simulink model "atrias_HW_boom_nmSt_kinSw_v4"  (R2015a)
settings: Solver=ode4  StartTime=0.0  StopTime=inf  FixedStep=sample_time  RelTol=1e-3
values from neighbouring files (symbols this model uses):
  control_start_time = 15    [setParams.m]
  flag_CtrlMode = 0    [setParams.m]
  kinSw_alpha_start = 130*pi/180    (= 2.26892802759)    [setParams.m]
  kinSw_alpha_tgt = 70*pi/180    (= 1.2217304764)    [setParams.m]
  kinSw_t_start = 0.5    [setParams.m]
  poser_LLegAlp = (initial_l_leg_angle -pi/2)*180/pi    (= 105)    [setParams.m]
  poser_LLegLen = initial_l_leg_length    (= 0.8)    [setParams.m]
  poser_RLegAlp = (initial_r_leg_angle -pi/2)*180/pi    (= 75)    [setParams.m]
  poser_RLegLen = initial_r_leg_length    (= 0.8)    [setParams.m]
  tune_kinSw_alpha_start = kinSw_alpha_start*180/pi    (= 130)    [setParams.m]
  tune_kinSw_alpha_tgt = kinSw_alpha_tgt*180/pi    (= 70)    [setParams.m]
  tune_kinSw_gClr_tgt = kinSw_gClr    (= 0.15)    [setParams.m]
  tune_kinSw_gH_tgt = kinSw_gH_tgt    (= -0.01)    [setParams.m]
  tune_M1_G = 9.5    [setParams.m]
  tune_M3_0 = CtrlPar_theta0*180/pi    [setParams.m]
  tune_M3_D = St_GainDTh_HFL*5    [setParams.m]
  tune_M3_P = St_GainTh_HFL*5    [setParams.m]
  tune_M4_G = 1    [setParams.m]
undefined symbols (not defined in the file or in its folder): A1_notch_f1, A2_notch_f1, A_kalman_fourbar_gear, A_lpf_dtau, B1_lpf_dtau, B1_notch_f1, B2_lpf_dtau, B2_notch_f1, B_kalman_fourbar_gear, boom_mount_angle, boom_mount_to_center_diagonal, c_jointstop, C_kalman_fourbar_gear, contactThr, d_vertical_com, delta_phi_max, delta_phi_max_buffer, delta_phi_max_dropoff, delta_phi_min, Discrete, FmaxBFSH, FmaxGLU, FmaxHAM, FmaxHFL, FmaxRF, FmaxVAS, FPCtrlPar, g, gain_nodes_sea_torque, HIP_MTR_MAX_CONT_TORQUE, initial_dx_estimate, j_motor, k_leg_spring, K_notch_f1, k_sea, kalman_load_to_deflect_transmission, kd_lateral, kd_motor, kd_shin_max, kd_shin_min, kd_splay_max, kd_splay_min, kd_thigh_max, kd_thigh_min, kp_lateral, kp_motor, kp_sea_torque, kp_shin_max, kp_shin_min, kp_splay_max, kp_splay_min, kp_thigh_max, kp_thigh_min, l_boom, l_seg, l_v, lateral_motor_efficiency, lateral_offset, lateral_target_angle_right, lateral_transition_force ... (+123)
libraries: simulink_extras x28, simulink x11, ctrlSharedLib x4
(part 1 of 8)
settings Model: CovSFcnEnable=off  Creator=wmartin  LastModifiedBy=smsong
settings SolverCC: EnableConcurrentExecution=on
settings DataIOCC: LimitDataPoints=off  MaxDataPoints=1000000000  SaveFormat=StructureWithTime  SignalLogging=off  DSMLogging=off  VisualizeSimOutput=off
settings OptimizationCC: BlockReduction=off  OptimizeBlockIOStorage=off  BufferReuse=off  GlobalBufferReuse=off  ExpressionFolding=off  ExpressionDepthLimit=2147483647  LocalBlockOutputs=off  SimCompilerOptimization=on
settings DebuggingCC: UnderspecifiedInitializationDetection=Classic  MergeDetectMultiDrivingBlocksExec=none  SolverPrmCheckMsg=warning  StateNameClashWarn=warning
settings HardwareCC: ProdIntDivRoundTo=Zero  ProdEndianess=LittleEndian  ProdLongLongMode=on  ProdHWDeviceType=Generic->32-bit x86 compatible
settings ModelReferenceCC: UpdateModelReferenceTargets=IfOutOfDate  ModelReferenceNumInstancesAllowed=Single  ModelReferenceMinAlgLoopOccurrences=on
settings RTWCC: SystemTargetFile=slrt.tlc  TemplateMakefile=slrt_default_tmf  Description=Simulink Real-Time  RTWVerbose=off  RTWCompilerOptimization=on
settings CodeAppCC: MaxIdLength=256
settings SimulinkRealTimeCC: GeneratePreprocessorConditionals=Disable all  RL32LogBufSizeModifier=1e8

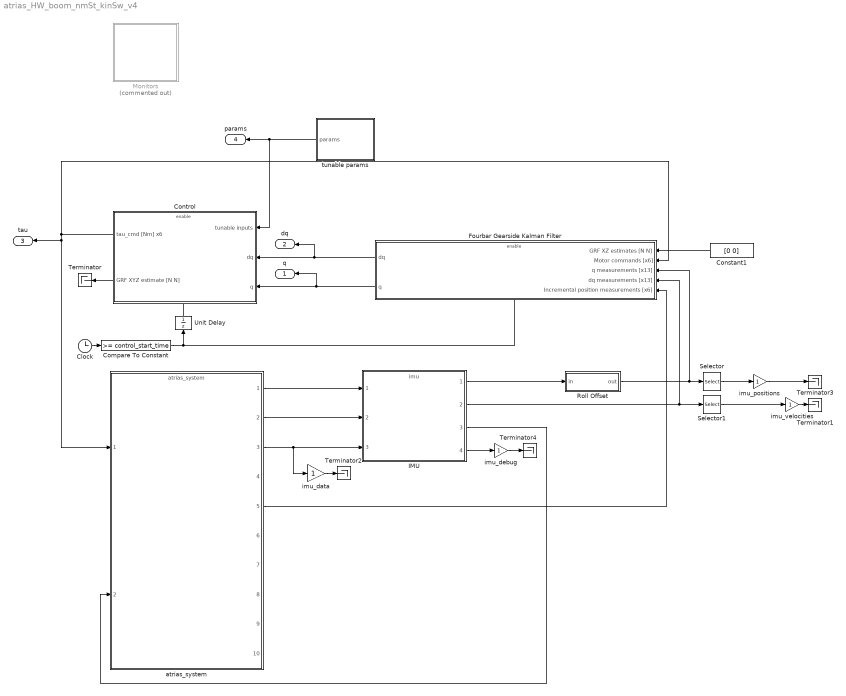
== system atrias_HW_boom_nmSt_kinSw_v4 ==
  Clock : Clock
  Compare To Constant : simulink/Logic and Bit Operations/Compare To Constant  relop=>=  const=control_start_time  OutDataTypeStr=boolean
  Constant1 : Constant  Value=[0 0]
  Control : Subsystem
  Fourbar Gearside Kalman Filter : Subsystem
  IMU : ModelReference  ModelNameDialog=imu  SimulationMode=Normal  ModelReferenceVersion=1.2453  CopyOfModelName=imu  DefaultDataLogging=on
  Monitors : Subsystem  Commented=on
  Roll Offset : Subsystem
  Selector : Selector  InputPortWidth=13  Indices=[11 12 13]
  Selector1 : Selector  InputPortWidth=13  Indices=[11 12 13]
  Terminator{,1..4} (5 alike) : Terminator
  Unit Delay : UnitDelay  SampleTime=-1
  atrias_system : ModelReference  ModelNameDialog=atrias_system  SimulationMode=Normal  ModelReferenceVersion=1.2798  CopyOfModelName=atrias_system  DefaultDataLogging=on
  imu_data : Gain
  imu_debug : Gain
  imu_positions : Gain
  imu_velocities : Gain
  tunable params : Subsystem
  q : Outport
  dq : Outport  Port=2
  tau : Outport  Port=3
  params : Outport  Port=4
  wires:
  Clock/1 -> Compare To Constant/1
  Compare To Constant/1 -> Fourbar Gearside Kalman Filter/Enable, Unit Delay/1
  imu_data/1 -> Terminator2/1
  imu_velocities/1 -> Terminator1/1
  imu_positions/1 -> Terminator3/1
  imu_debug/1 -> Terminator4/1
  IMU/4 -> imu_debug/1
  Selector/1 -> imu_positions/1
  Selector1/1 -> imu_velocities/1
  atrias_system/1 -> IMU/1
  IMU/2 -> Fourbar Gearside Kalman Filter/4(dq measurements [x13]), Selector1/1
  IMU/1 -> Roll Offset/1(in)
  Control/1(tau_cmd [Nm] x6) -> atrias_system/1, tau/1, Fourbar Gearside Kalman Filter/2(Motor commands [x6])
  atrias_system/2 -> IMU/2
  atrias_system/3 -> imu_data/1, IMU/3
  IMU/3 -> atrias_system/2
  Unit Delay/1 -> Control/Enable
  Control/2(GRF XYZ estimate [N N]) -> Terminator/1
  Fourbar Gearside Kalman Filter/1(dq) -> dq/1, Control/2(dq)
  Fourbar Gearside Kalman Filter/2(q) -> q/1, Control/3(q)
  atrias_system/5 -> Fourbar Gearside Kalman Filter/5(Incremental position measurements [x6])
  Constant1/1 -> Fourbar Gearside Kalman Filter/1(GRF XZ estimates [N N])
  Roll Offset/1(out) -> Fourbar Gearside Kalman Filter/3(q measurements [x13]), Selector/1
  tunable params/1(params) -> params/1, Control/1(tunable inputs)

== system atrias_HW_boom_nmSt_kinSw_v4/Control ==
  tunable inputs : Inport
  dq : Inport  Port=2
  q : Inport  Port=3
  Enable : EnablePort  StatesWhenEnabling=reset  PropagateVarSize=During execution
  Actuator Control : Subsystem
  Behavior Control : Subsystem
  Control Switch : Subsystem
  Poser : Subsystem
  Tunable Control Parameters : Subsystem
  tau_cmd [Nm] x6 : Outport  InitialOutput=[0 0 0 0 0 0]
  GRF XYZ estimate [N N] : Outport  Port=2  InitialOutput=[0 0 0]
  wires:
  q/1 -> Behavior Control/2(q [rad] x13), Actuator Control/4(q)
  dq/1 -> Behavior Control/1(dq [rad/s] x13), Actuator Control/5(dq)
  Actuator Control/1(tau_cmd [Nm] x6) -> tau_cmd [Nm] x6/1
  Behavior Control/4(GRF XYZ estimates [N N N]) -> GRF XYZ estimate [N N]/1
  tunable inputs/1 -> Tunable Control Parameters/1(tunable inputs)
  Control Switch/3(Force / Position Control [1/0] x4) -> Actuator Control/3(Enable SEA Control [1/0] x4)
  Control Switch/2(SEA Torque Velocity Command [Nm] x4) -> Actuator Control/2(Desired SEA Torque Velocity [Nm] x4)
  Control Switch/1(Motor Torque Command [Nm] x6) -> Actuator Control/1(Desired Torque [Nm] x6)
  Poser/1(Motor Torque Command [Nm] x6) -> Control Switch/1(Pose Comm [Nm] x6)
  Poser/2(SEA Torque Velocity Command [Nm] x4) -> Control Switch/2(Pose Comm [Nm] x4)
  Poser/3(Force / Position Control [1/0] x4) -> Control Switch/3(Pose Comm [1/0] x4)
  Behavior Control/1(Motor Torque Command [Nm] x6) -> Control Switch/4(NM Comm [Nm] x6)
  Behavior Control/2(SEA Torque Velocity Command [Nm] x4) -> Control Switch/5(NM Comm [Nm] x4)
  Behavior Control/3(Force / Position Control [1/0] x4) -> Control Switch/6(NM Comm [1/0] x4)

== system atrias_HW_boom_nmSt_kinSw_v4/Fourbar Gearside Kalman Filter ==
  note: Order:
      | rightBack
      | rightFront
      | leftBack
      | leftFront
  GRF XZ estimates [N N] : Inport  SampleTime=sample_time
  Motor commands [x6] : Inport  Port=2  SampleTime=sample_time
  q measurements [x13] : Inport  Port=3  SampleTime=sample_time
  dq measurements [x13] : Inport  Port=4  SampleTime=sample_time
  Incremental position measurements [x6] : Inport  Port=5  SampleTime=sample_time
  Enable : EnablePort  ShowOutputPort=on
  Covariance Estimates : MATLAB Function  TreatAsAtomicUnit=on
  Demux{,1..4} (5 alike) : Demux
  Demux{5..8} (4 alike) : Demux  Outputs=2
  External Trunk Torque Estimate : MATLAB Function  TreatAsAtomicUnit=on
  Fourbar Gear Kalman Filter {1..4} (4 alike) : ctrlSharedLib/Kalman Filter  TimeDomain=Discrete-Time  UseCurrentEstimator=on  ModelSource=Individual A, B, C, D matrices  ModelSourceVariable=A_kf  A=A_kalman_fourbar_gear  B=B_kalman_fourbar_gear  C=C_kalman_fourbar_gear  D=0  NumberOfStates=2  NumberOfInputs=1  NumberOfOutputs=2  InitialEstimateSource=Input port  X0=initial_dx_estimate  P0=P0_kalman_transverse  UseK=off  UseGH=on  NumberOfProcessNoiseInputs=1  G=G_kalman_fourbar_gear  TimeInvariantG=on  H=0  TimeInvariantH=on  Q=1  TimeInvariantQ=off  R=1  TimeInvariantR=off  N=0  TimeInvariantN=on  AddInputPort=on  AddEnablePort=off  ExternalReset=Either  OutputEstimatedY=off  OutputP=on  Ts=sample_time
  Mux{,3,7..9,11,13,15,17..18} (10 alike) : Mux  Inputs=2
  Mux{1,4..6,16} (5 alike) : Mux
  Mux{2,10,12,14} (4 alike) : Mux  Inputs=3
  P0_kalman_fourbar_gear{,1..3} (4 alike) : Constant  Value=P0_kalman_fourbar_gear
  Selector : Selector  InputPortWidth=17  Indices=[1 14 3 15 5 16 7 17 9 10 11 12 13]
  Selector1 : Selector  InputPortWidth=17  Indices=[1 14 3 15 5 16 7 17 9 10 11 12 13]
  Spring Stiffness 1 : Gain  Gain=k_sea
  Spring Stiffness 2 : Gain  Gain=1/LEG_MTR_GEAR_RATIO
  Sum : Sum  Inputs=-|+
  Terminator : Terminator
  Terminator1 : Terminator
  Terminator2 : Terminator
  Unit Delay{,1..9} (10 alike) : UnitDelay  SampleTime=-1
  Zero-Order Hold : ZeroOrderHold  SampleTime=sample_time
  eigen values 1 : MATLAB Function  TreatAsAtomicUnit=on
  eigen values 2 : MATLAB Function  TreatAsAtomicUnit=on
  eigen values 3 : MATLAB Function  TreatAsAtomicUnit=on
  "eigen values4 " : MATLAB Function  TreatAsAtomicUnit=on
  kalman_filtered_position : Gain
  kalman_filtered_velocity : Gain
  kalman_uncertainty : Gain
  select absolute relative gear position : Selector  InputPortWidth=13  Indices=[2 4 6 8]
  select absolute relative gear velocity : Selector  InputPortWidth=13  Indices=[2 4 6 8]
  select absolute relative load position : Selector  InputPortWidth=13  Indices=[2 4 6 8]
  select fourbar motors : Selector  InputPortWidth=6  Indices=[1 2 3 4]
  select incremental relative gear position : Selector  InputPortWidth=6  Indices=[1 2 3 4]
  select torso pitch : Selector  InputPortWidth=13  Indices=[13]
  select_position{1,3,5,7} (4 alike) : Selector  NumberOfDimensions=2  InputPortWidth=2  IndexOptions=Index vector (dialog),Index vector (dialog)  Indices=[1],[1]  OutputSizes=1,1
  dq : Outport
  q : Outport  Port=2
  wires:
  select incremental relative gear position/1 -> Demux/1
  q measurements [x13]/1 -> select absolute relative gear position/1, Mux17/1, select absolute relative load position/1, select torso pitch/1
  Incremental position measurements [x6]/1 -> select incremental relative gear position/1
  Motor commands [x6]/1 -> Unit Delay8/1
  select fourbar motors/1 -> Spring Stiffness 2/1
  P0_kalman_fourbar_gear/1 -> Fourbar Gear Kalman Filter 1/4
  Mux/1 -> Fourbar Gear Kalman Filter 1/3
  select absolute relative gear velocity/1 -> Demux3/1
  dq measurements [x13]/1 -> Mux18/1, select absolute relative gear velocity/1
  Demux3/1 -> Mux/2
  GRF XZ estimates [N N]/1 -> Unit Delay9/1
  Spring Stiffness 1/1 -> Demux4/1, External Trunk Torque Estimate/3(spring_torque), Covariance Estimates/1(spring_torque)
  Fourbar Gear Kalman Filter 1/1 -> Unit Delay/1
  Demux5/1 -> Mux1/1, Mux5/1
  Mux1/1 -> Sum/2, Mux17/2, kalman_filtered_position/1
  select absolute relative load position/1 -> Sum/1
  Sum/1 -> Spring Stiffness 1/1
  External Trunk Torque Estimate/1(tau_trunk) -> Mux2/3, Mux10/3, Mux12/3, Mux14/3
  Demux4/1 -> Mux2/1
  Demux2/1 -> Mux2/2
  Mux2/1 -> Fourbar Gear Kalman Filter 1/1
  Demux/1 -> Mux3/2
  Demux1/1 -> Mux3/1, Mux/1
  Mux3/1 -> Fourbar Gear Kalman Filter 1/2
  Fourbar Gear Kalman Filter 1/2 -> Unit Delay1/1
  Mux4/1 -> Covariance Estimates/4(state_uncertainty)
  select absolute relative gear position/1 -> Covariance Estimates/2(absolute_gear), Demux1/1
  Mux5/1 -> Covariance Estimates/3(current_position_estimate)
  Covariance Estimates/1(Q1) -> Fourbar Gear Kalman Filter 1/6
  Covariance Estimates/2(R1) -> Fourbar Gear Kalman Filter 1/7
  select torso pitch/1 -> External Trunk Torque Estimate/4(torso_pitch)
  select_position1/1 -> Mux4/1
  P0_kalman_fourbar_gear1/1 -> Fourbar Gear Kalman Filter 2/4
  Fourbar Gear Kalman Filter 2/1 -> Unit Delay2/1
  Fourbar Gear Kalman Filter 2/2 -> Unit Delay3/1
  P0_kalman_fourbar_gear2/1 -> Fourbar Gear Kalman Filter 3/4
  Fourbar Gear Kalman Filter 3/1 -> Unit Delay4/1
  Fourbar Gear Kalman Filter 3/2 -> Unit Delay5/1
  P0_kalman_fourbar_gear3/1 -> Fourbar Gear Kalman Filter 4/4
  Fourbar Gear Kalman Filter 4/1 -> Unit Delay6/1
  Fourbar Gear Kalman Filter 4/2 -> Unit Delay7/1
  Covariance Estimates/3(Q2) -> Fourbar Gear Kalman Filter 2/6
  Covariance Estimates/5(Q3) -> Fourbar Gear Kalman Filter 3/6
  Covariance Estimates/7(Q4) -> Fourbar Gear Kalman Filter 4/6
  Covariance Estimates/4(R2) -> Fourbar Gear Kalman Filter 2/7
  Covariance Estimates/6(R3) -> Fourbar Gear Kalman Filter 3/7
  Covariance Estimates/8(R4) -> Fourbar Gear Kalman Filter 4/7
  select_position3/1 -> Mux4/2
  select_position5/1 -> Mux4/3
  select_position7/1 -> Mux4/4
  Demux6/1 -> Mux5/2, Mux1/2
  Demux7/1 -> Mux1/3, Mux5/3
  Demux8/1 -> Mux1/4, Mux5/4
  kalman_filtered_position/1 -> Terminator/1
  Enable/1 -> Zero-Order Hold/1
  Mux7/1 -> Fourbar Gear Kalman Filter 2/3
  Mux8/1 -> Fourbar Gear Kalman Filter 3/3
  Mux9/1 -> Fourbar Gear Kalman Filter 4/3
  Mux10/1 -> Fourbar Gear Kalman Filter 2/1
  Mux11/1 -> Fourbar Gear Kalman Filter 2/2
  Mux13/1 -> Fourbar Gear Kalman Filter 3/2
  Mux12/1 -> Fourbar Gear Kalman Filter 3/1
  Mux15/1 -> Fourbar Gear Kalman Filter 4/2
  Mux14/1 -> Fourbar Gear Kalman Filter 4/1
  Demux3/2 -> Mux7/2
  Demux3/3 -> Mux8/2
  Demux3/4 -> Mux9/2
  Demux1/2 -> Mux7/1, Mux11/1
  Demux1/3 -> Mux13/1, Mux8/1
  Demux1/4 -> Mux9/1, Mux15/1
  Demux/2 -> Mux11/2
  Demux/3 -> Mux13/2
  Demux/4 -> Mux15/2
  Demux4/2 -> Mux10/1
  Demux4/3 -> Mux12/1
  Demux4/4 -> Mux14/1
  Demux2/2 -> Mux10/2
  Demux2/3 -> Mux12/2
  Demux2/4 -> Mux14/2
  kalman_uncertainty/1 -> Terminator1/1
  Mux6/1 -> kalman_uncertainty/1
  kalman_filtered_velocity/1 -> Terminator2/1
  Mux16/1 -> Mux18/2, kalman_filtered_velocity/1
  Demux5/2 -> Mux16/1
  Demux6/2 -> Mux16/2
  Demux7/2 -> Mux16/3
  Demux8/2 -> Mux16/4
  Zero-Order Hold/1 -> Fourbar Gear Kalman Filter 4/5, Fourbar Gear Kalman Filter 3/5, Fourbar Gear Kalman Filter 2/5, Fourbar Gear Kalman Filter 1/5
  Unit Delay1/1 -> eigen values 1/1(Z), select_position1/1
  Unit Delay3/1 -> eigen values 2/1(Z), select_position3/1
  Unit Delay4/1 -> Demux7/1
  Unit Delay7/1 -> "eigen values4 "/1(Z), select_position7/1
  Unit Delay6/1 -> Demux8/1
  Spring Stiffness 2/1 -> Demux2/1, External Trunk Torque Estimate/2(rotor_torque)
  Unit Delay5/1 -> eigen values 3/1(Z), select_position5/1
  eigen values 1/1(E) -> Mux6/1
  eigen values 2/1(E) -> Mux6/2
  eigen values 3/1(E) -> Mux6/3
  "eigen values4 "/1(E) -> Mux6/4
  Unit Delay/1 -> Demux5/1
  Unit Delay2/1 -> Demux6/1
  Mux17/1 -> Selector/1
  Selector/1 -> q/1
  Selector1/1 -> dq/1
  Mux18/1 -> Selector1/1
  Unit Delay8/1 -> select fourbar motors/1
  Unit Delay9/1 -> External Trunk Torque Estimate/1(grf_xz)

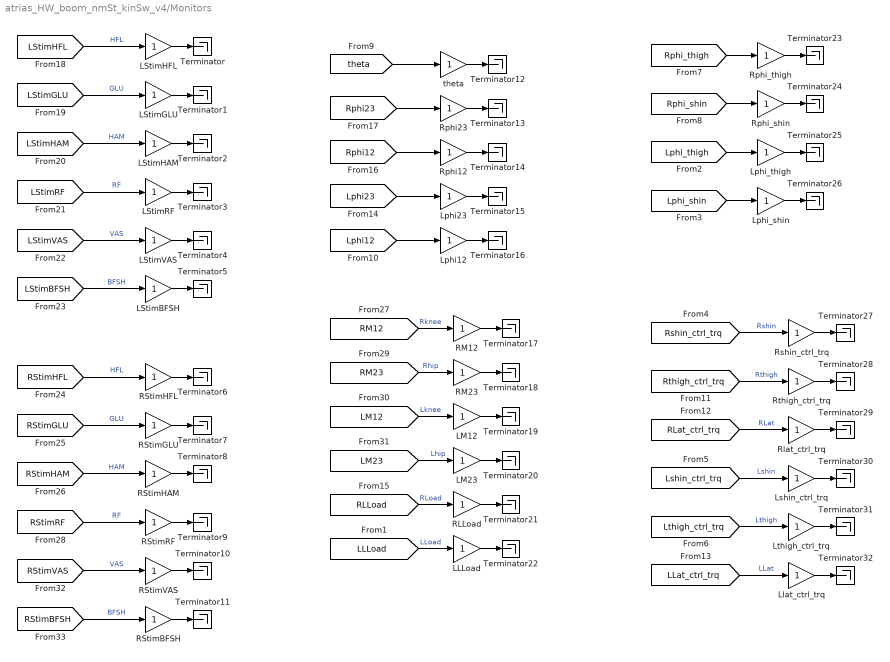
== system atrias_HW_boom_nmSt_kinSw_v4/Monitors ==
  LLLoad : Gain
  LM12 : Gain
  LM23 : Gain
  LStimBFSH : Gain
  LStimGLU : Gain
  LStimHAM : Gain
  LStimHFL : Gain
  LStimRF : Gain
  LStimVAS : Gain
  Llat_ctrl_trq : Gain
  Lphi12 : Gain
  Lphi23 : Gain
  Lphi_shin : Gain
  Lphi_thigh : Gain
  Lshin_ctrl_trq : Gain
  Lthigh_ctrl_trq : Gain
  RLLoad : Gain
  RM12 : Gain
  RM23 : Gain
  RStimBFSH : Gain
  RStimGLU : Gain
  RStimHAM : Gain
  RStimHFL : Gain
  RStimRF : Gain
  RStimVAS : Gain
  Rlat_ctrl_trq : Gain
  Rphi12 : Gain
  Rphi23 : Gain
  Rphi_shin : Gain
  Rphi_thigh : Gain
  Rshin_ctrl_trq : Gain
  Rthigh_ctrl_trq : Gain
  Terminator{,1..32} (33 alike) : Terminator
  theta : Gain
  wires:
  [Rphi_thigh] -> Rphi_thigh/1
  [Rphi_shin] -> Rphi_shin/1
  [Lphi_thigh] -> Lphi_thigh/1
  [Lphi_shin] -> Lphi_shin/1
  [theta] -> theta/1
  [Rphi12] -> Rphi12/1
  [Lphi23] -> Lphi23/1
  [Lphi12] -> Lphi12/1
  [Rphi23] -> Rphi23/1
  [Rshin_ctrl_trq] -> Rshin_ctrl_trq/1  "Rshin"
  [Rthigh_ctrl_trq] -> Rthigh_ctrl_trq/1  "Rthigh"
  [RLat_ctrl_trq] -> Rlat_ctrl_trq/1  "RLat"
  [Lshin_ctrl_trq] -> Lshin_ctrl_trq/1  "Lshin"
  [Lthigh_ctrl_trq] -> Lthigh_ctrl_trq/1  "Lthigh"
  [LLat_ctrl_trq] -> Llat_ctrl_trq/1  "LLat"
  [LM12] -> LM12/1  "Lknee"
  [LM23] -> LM23/1  "Lhip"
  [RM23] -> RM23/1  "Rhip"
  [RM12] -> RM12/1  "Rknee"
  [LLLoad] -> LLLoad/1  "LLoad"
  [RLLoad] -> RLLoad/1  "RLoad"
  [LStimHFL] -> LStimHFL/1  "HFL"
  [LStimGLU] -> LStimGLU/1  "GLU"
  [LStimHAM] -> LStimHAM/1  "HAM"
  [LStimRF] -> LStimRF/1  "RF"
  [LStimVAS] -> LStimVAS/1  "VAS"
  [LStimBFSH] -> LStimBFSH/1  "BFSH"
  [RStimHFL] -> RStimHFL/1  "HFL"
  [RStimGLU] -> RStimGLU/1  "GLU"
  [RStimHAM] -> RStimHAM/1  "HAM"
  [RStimRF] -> RStimRF/1  "RF"
  [RStimVAS] -> RStimVAS/1  "VAS"
  [RStimBFSH] -> RStimBFSH/1  "BFSH"
  LStimHFL/1 -> Terminator/1
  LStimGLU/1 -> Terminator1/1
  LStimHAM/1 -> Terminator2/1
  LStimRF/1 -> Terminator3/1
  LStimVAS/1 -> Terminator4/1
  LStimBFSH/1 -> Terminator5/1
  RStimHFL/1 -> Terminator6/1
  RStimGLU/1 -> Terminator7/1
  RStimHAM/1 -> Terminator8/1
  RStimRF/1 -> Terminator9/1
  RStimVAS/1 -> Terminator10/1
  RStimBFSH/1 -> Terminator11/1
  theta/1 -> Terminator12/1
  Rphi23/1 -> Terminator13/1
  Rphi12/1 -> Terminator14/1
  Lphi23/1 -> Terminator15/1
  Lphi12/1 -> Terminator16/1
  RM12/1 -> Terminator17/1
  RM23/1 -> Terminator18/1
  LM12/1 -> Terminator19/1
  LM23/1 -> Terminator20/1
  RLLoad/1 -> Terminator21/1
  LLLoad/1 -> Terminator22/1
  Rphi_thigh/1 -> Terminator23/1
  Rphi_shin/1 -> Terminator24/1
  Lphi_thigh/1 -> Terminator25/1
  Lphi_shin/1 -> Terminator26/1
  Rshin_ctrl_trq/1 -> Terminator27/1
  Rthigh_ctrl_trq/1 -> Terminator28/1
  Rlat_ctrl_trq/1 -> Terminator29/1
  Lshin_ctrl_trq/1 -> Terminator30/1
  Lthigh_ctrl_trq/1 -> Terminator31/1
  Llat_ctrl_trq/1 -> Terminator32/1

== system atrias_HW_boom_nmSt_kinSw_v4/Roll Offset ==
  in : Inport
  11 : Selector  InputPortWidth=13  Indices=[11]
  Constant2 : Constant  Value=boom_mount_angle
  Mux : Mux  Inputs=2
  Sum : Sum  Inputs=++|
  except 11 : Selector  InputPortWidth=13  Indices=[1 2 3 4 5 6 7 8 9 10 12 13]
  remap : Selector  InputPortWidth=13  Indices=[1 2 3 4 5 6 7 8 9 10 13 11 12]
  out : Outport
  wires:
  except 11/1 -> Mux/1
  Mux/1 -> remap/1
  Constant2/1 -> Sum/1
  in/1 -> 11/1, except 11/1
  Sum/1 -> Mux/2
  11/1 -> Sum/2
  remap/1 -> out/1

== system atrias_HW_boom_nmSt_kinSw_v4/tunable params ==
  note: do not forget to set the params of the low pass filters!!
  Constant1 : Constant  Value=tune_M4_G
  Constant11 : Constant  Value=tune_M1_G
  Constant12 : Constant  Value=tune_M3_0
  Constant18 : Constant  Value=tune_M3_D
  Constant20 : Constant  Value=tune_M3_P
  Constant28 : Constant  Value=poser_RLegLen
  Constant29 : Constant  Value=poser_RLegAlp
  Constant30 : Constant  Value=poser_LLegLen
  Constant31 : Constant  Value=poser_LLegAlp
  Constant36 : Constant  Value=tune_kinSw_alpha_start
  Constant37 : Constant  Value=tune_kinSw_alpha_tgt
  Constant38 : Constant  Value=tune_kinSw_gH_tgt
  Constant39 : Constant  Value=tune_kinSw_gClr_tgt
  Mux2 : Mux  Inputs=13
  low pass filter : simulink_extras/Additional Linear/Transfer Fcn (with initial outputs)  N=[1]  D="[.5  1]"  Y0=tune_M1_G  U0=tune_M1_G
      settings: AttributesFormatString=pre-activation: %<Y0>
  low pass filter1 : simulink_extras/Additional Linear/Transfer Fcn (with initial outputs)  N=[1]  D="[.5  1]"  Y0=tune_M3_0  U0=tune_M3_0
      settings: AttributesFormatString=pre-activation: %<Y0>
  low pass filter10 : simulink_extras/Additional Linear/Transfer Fcn (with initial outputs)  N=[1]  D="[.5  1]"  Y0=poser_LLegLen  U0=poser_LLegLen
      settings: AttributesFormatString=pre-activation: %<Y0>
  low pass filter11 : simulink_extras/Additional Linear/Transfer Fcn (with initial outputs)  N=[1]  D="[.5  1]"  Y0=poser_LLegAlp  U0=poser_LLegAlp
      settings: AttributesFormatString=pre-activation: %<Y0>
  low pass filter12 : simulink_extras/Additional Linear/Transfer Fcn (with initial outputs)  N=[1]  D="[.5  1]"  Y0=tune_M4_G  U0=tune_M4_G
      settings: AttributesFormatString=pre-activation: %<Y0>
  low pass filter2 : simulink_extras/Additional Linear/Transfer Fcn (with initial outputs)  N=[1]  D="[.5  1]"  Y0=tune_M3_P  U0=tune_M3_P
      settings: AttributesFormatString=pre-activation: %<Y0>
  low pass filter3 : simulink_extras/Additional Linear/Transfer Fcn (with initial outputs)  N=[1]  D="[.5  1]"  Y0=tune_M3_D  U0=tune_M3_D
      settings: AttributesFormatString=pre-activation: %<Y0>
  low pass filter4 : simulink_extras/Additional Linear/Transfer Fcn (with initial outputs)  N=[1]  D="[.5  1]"  Y0=tune_kinSw_alpha_start  U0=tune_kinSw_alpha_start
      settings: AttributesFormatString=pre-activation: %<Y0>
  low pass filter5 : simulink_extras/Additional Linear/Transfer Fcn (with initial outputs)  N=[1]  D="[.5  1]"  Y0=tune_kinSw_alpha_tgt  U0=tune_kinSw_alpha_tgt
      settings: AttributesFormatString=pre-activation: %<Y0>
  low pass filter6 : simulink_extras/Additional Linear/Transfer Fcn (with initial outputs)  N=[1]  D="[.5  1]"  Y0=tune_kinSw_gH_tgt  U0=tune_kinSw_gH_tgt
      settings: AttributesFormatString=pre-activation: %<Y0>
  low pass filter7 : simulink_extras/Additional Linear/Transfer Fcn (with initial outputs)  N=[1]  D="[.5  1]"  Y0=tune_kinSw_gClr_tgt  U0=tune_kinSw_gClr_tgt
      settings: AttributesFormatString=pre-activation: %<Y0>
  low pass filter8 : simulink_extras/Additional Linear/Transfer Fcn (with initial outputs)  N=[1]  D="[.5  1]"  Y0=poser_RLegLen  U0=poser_RLegLen
      settings: AttributesFormatString=pre-activation: %<Y0>
  low pass filter9 : simulink_extras/Additional Linear/Transfer Fcn (with initial outputs)  N=[1]  D="[.5  1]"  Y0=poser_RLegAlp  U0=poser_RLegAlp
      settings: AttributesFormatString=pre-activation: %<Y0>
  params : Outport
  wires:
  Mux2/1 -> params/1
  Constant18/1 -> low pass filter3/1
  Constant11/1 -> low pass filter/1
  Constant36/1 -> low pass filter4/1
  Constant37/1 -> low pass filter5/1
  Constant12/1 -> low pass filter1/1
  Constant38/1 -> low pass filter6/1
  Constant39/1 -> low pass filter7/1
  Constant20/1 -> low pass filter2/1
  low pass filter/1 -> Mux2/1
  low pass filter1/1 -> Mux2/2
  low pass filter2/1 -> Mux2/3
  low pass filter3/1 -> Mux2/4
  low pass filter4/1 -> Mux2/6
  low pass filter5/1 -> Mux2/7
  low pass filter6/1 -> Mux2/8
  low pass filter7/1 -> Mux2/9
  Constant28/1 -> low pass filter8/1
  low pass filter8/1 -> Mux2/10
  Constant29/1 -> low pass filter9/1
  low pass filter9/1 -> Mux2/11
  Constant30/1 -> low pass filter10/1
  low pass filter10/1 -> Mux2/12
  Constant31/1 -> low pass filter11/1
  low pass filter11/1 -> Mux2/13
  Constant1/1 -> low pass filter12/1
  low pass filter12/1 -> Mux2/5

== system atrias_HW_boom_nmSt_kinSw_v4/Control/Actuator Control ==
  note: Order:
      | backR
      | frontR
      | backL
      | frontL
  note: Motor Order:
      |
      | backR
      | frontR
      | latR
      | backL
      | frontL
      | latL
  Desired Torque [Nm] x6 : Inport  OutDataTypeStr=double  PortDimensions=6  SampleTime=sample_time
  Desired SEA Torque Velocity [Nm] x4 : Inport  Port=2  OutDataTypeStr=double  PortDimensions=4  SampleTime=sample_time
  Enable SEA Control [1/0] x4 : Inport  Port=3  OutDataTypeStr=boolean  PortDimensions=4  SampleTime=sample_time
  q : Inport  Port=4  OutDataTypeStr=double  PortDimensions=13  SampleTime=sample_time
  dq : Inport  Port=5  OutDataTypeStr=double  PortDimensions=13  SampleTime=sample_time
  Activate SEA Control : Subsystem
  Antiresonance Compensation : Subsystem
  Hip Motor Efficiency Compensation : Gain  Gain=1/lateral_motor_efficiency
  Leg Motor Efficiency Compensation : Gain  Gain=1/sagittal_motor_efficiency
  Mux{1..2,4..5} (4 alike) : Mux
  Mux3 : Mux  Inputs=2
  SEA Control Toggle : Subsystem
  SEA Controller (Torque) : Subsystem
  Selector12 : Selector  InputPortWidth=13  Indices=[5 6]
  Selector13 : Selector  InputPortWidth=13  Indices=[7 8]
  Selector15 : Selector  InputPortWidth=13  Indices=[1 2]
  Selector16 : Selector  InputPortWidth=13  Indices=[3 4]
  Selector{17..20,25..28} (8 alike) : Selector  InputPortWidth=2  Indices=[1]
  Selector2 : Selector  InputPortWidth=13  Indices=[5 6]
  Selector{21..24,29..32} (8 alike) : Selector  InputPortWidth=2  Indices=[2]
  Selector3 : Selector  InputPortWidth=6  Indices=[3 6]
  Selector33 : Selector  InputPortWidth=6  Indices=[1 2 4 5]
  Selector4 : Selector  InputPortWidth=13  Indices=[7 8]
  Selector6 : Selector  InputPortWidth=13  Indices=[1 2]
  Selector7 : Selector  InputPortWidth=13  Indices=[3 4]
  Selector8 : Selector  InputPortWidth=6  Indices=[1 2 5 3 4 6]
  Selector9 : Selector  InputPortWidth=6  Indices=[1 2 4 5]
  Terminator1 : Terminator
  Torque Limiter (outside) 1 : Saturate  UpperLimit=max_sagittal_unloaded_torque  LowerLimit=-max_sagittal_unloaded_torque
      settings: AttributesFormatString=Hi: %<UpperLimit>\nLo: %<LowerLimit>
  tau_desired_signals : Gain  Description=xPCTag(1)=tau_cmd_signal;
  tau_cmd [Nm] x6 : Outport  OutDataTypeStr=double  PortDimensions=6  SampleTime=0  InitialOutput=[0 0 0 0 0 0]
  wires:
  Selector3/1 -> Hip Motor Efficiency Compensation/1
  [dqFrontL] -> Selector32/1
  Selector29/1 -> Mux5/1
  Selector18/1 -> Mux1/2
  Selector19/1 -> Mux1/3
  Selector2/1 -> [qBackL]
  Selector15/1 -> [dqBackR]
  dq/1 -> Selector13/1, Selector15/1, Selector16/1, Selector12/1
  tau_desired_signals/1 -> Terminator1/1
  Selector7/1 -> [qFrontR]
  Torque Limiter (outside) 1/1 -> Activate SEA Control/3(Torque Signal [Nm] x4), SEA Control Toggle/3(tau_cmd)
  Desired Torque [Nm] x6/1 -> Selector33/1, Selector9/1, Selector3/1, tau_desired_signals/1
  Selector8/1 -> tau_cmd [Nm] x6/1
  Selector6/1 -> [qBackR]
  SEA Controller (Torque)/1(tau_cmd sagittal [Nm] x4) -> Activate SEA Control/1(SEA Control Signal [Nm] x4)
  SEA Controller (Torque)/2(tau_measured [Nm] x4) -> SEA Control Toggle/2(tau_measured)
  Activate SEA Control/1(Torque Command [Nm] x4) -> Leg Motor Efficiency Compensation/1
  q/1 -> Selector2/1, Selector7/1, Selector6/1, Selector4/1
  Selector16/1 -> [dqFrontR]
  Selector4/1 -> [qFrontL]
  Selector9/1 -> Antiresonance Compensation/1(Torque)
  [qBackL] -> Selector23/1
  Selector26/1 -> Mux4/2
  Selector30/1 -> Mux5/2
  Mux5/1 -> SEA Controller (Torque)/6(dphi_gear [rad/s] x4)
  Leg Motor Efficiency Compensation/1 -> Mux3/1
  Selector24/1 -> Mux2/4
  [qFrontR] -> Selector18/1
  [qFrontL] -> Selector20/1
  [qBackR] -> Selector21/1
  Antiresonance Compensation/1(Filtered Torque) -> Torque Limiter (outside) 1/1
  Selector13/1 -> [dqFrontL]
  Selector23/1 -> Mux2/3
  Mux1/1 -> SEA Controller (Torque)/1(phi_load [rad] x4)
  [dqFrontL] -> Selector28/1
  Desired SEA Torque Velocity [Nm] x4/1 -> SEA Controller (Torque)/4(dtau_des sagittal [Nm] x4)
  Selector25/1 -> Mux4/1
  Selector31/1 -> Mux5/3
  [dqBackL] -> Selector31/1
  Hip Motor Efficiency Compensation/1 -> Mux3/2
  Selector28/1 -> Mux4/4
  [qFrontL] -> Selector24/1
  Selector22/1 -> Mux2/2
  [dqFrontR] -> Selector30/1
  Selector32/1 -> Mux5/4
  Mux4/1 -> SEA Controller (Torque)/5(dphi_load [rad/s] x4)
  Mux3/1 -> Selector8/1
  [dqBackR] -> Selector29/1
  Selector27/1 -> Mux4/3
  [qFrontR] -> Selector22/1
  Selector21/1 -> Mux2/1
  [dqBackL] -> Selector27/1
  [dqBackR] -> Selector25/1
  Selector20/1 -> Mux1/4
  Selector17/1 -> Mux1/1
  [qBackR] -> Selector17/1
  [qBackL] -> Selector19/1
  Selector12/1 -> [dqBackL]
  Mux2/1 -> SEA Controller (Torque)/2(phi_gear [rad] x4)
  SEA Control Toggle/1(SEA Control on/off [1/0]) -> Activate SEA Control/2("SEA on/off [1/0] x4 ")
  Selector33/1 -> SEA Controller (Torque)/3(tau_des sagittal [Nm] x4)
  Enable SEA Control [1/0] x4/1 -> SEA Control Toggle/1(enable)
  [dqFrontR] -> Selector26/1

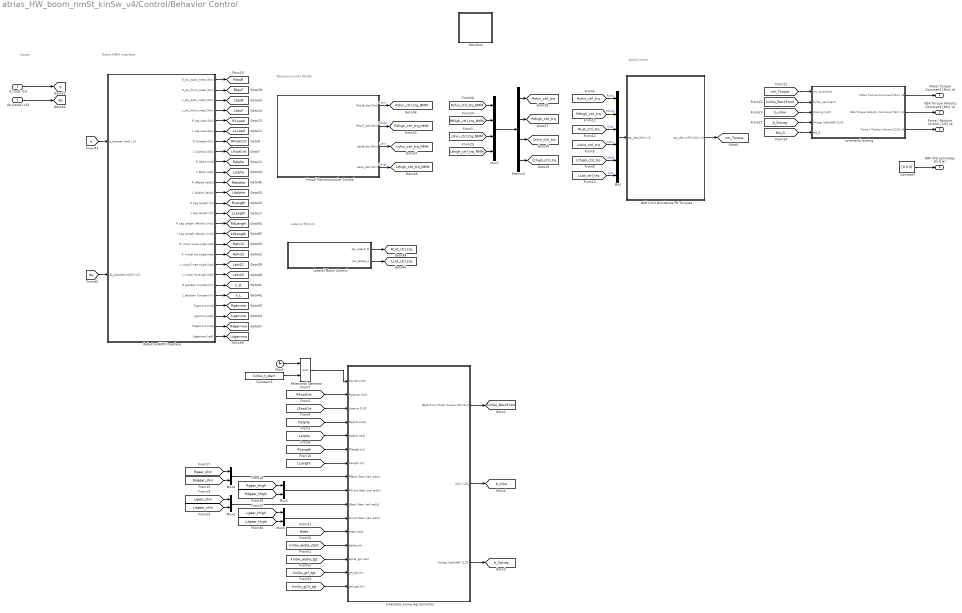
== system atrias_HW_boom_nmSt_kinSw_v4/Control/Behavior Control ==
  note: Robot-NMM Interface
  note: Inputs
  note: Neuromuscular Model
  note: Avoid Limits
  note: Lateral Motors
  dq [rad/s] x13 : Inport
  q [rad] x13 : Inport  Port=2
  Add Limit Avoidance PD Torques : Subsystem
  Clock : Clock
  Constant : Constant  Value=[0 0 0]
  Constant1 : Constant  Value=kinSw_t_start
  Demux3 : Demux
  Lateral Motor Control : Subsystem
  Monitors : Subsystem
  Mux : Mux  Inputs=6
  Mux{1..4} (4 alike) : Mux  Inputs=2
  Mux7 : Mux
  Relational Operator : RelationalOperator
  Robot-to-NMM Interface : Subsystem
  Virtual Neuromuscular Control : Subsystem  SystemSampleTime=sample_time
  command routing : Subsystem
  kinematic swing leg controller : Subsystem
  Motor Torque Command [Nm] x6 : Outport  OutputWhenDisabled=reset  InitialOutput=[0 0 0 0 0 0]
  SEA Torque Velocity Command [Nm] x4 : Outport  Port=2  OutputWhenDisabled=reset  InitialOutput=[0 0 0 0 0 0]
  Force / Position Control [1/0] x4 : Outport  Port=3  OutputWhenDisabled=reset  InitialOutput=[0 0 0 0 0 0]
  GRF XYZ estimates [N N N] : Outport  Port=4  OutputWhenDisabled=reset  InitialOutput=[0 0 0 0 0 0]
  tag scope: LFootCnt=global, LLLoad=global, LLat_ctrl_trq=global, LLength=global, Lalpha=global, LdLength=global, Ldalpha=global, Ldgamma=global, Lgamma=global, Lphi12=global, Lphi23=global, Lshin_ctrl_trq=global, Lshin_ctrl_trq_NMM=global, LtauB=global, LtauF=global, Lthigh_ctrl_trq=global, Lthigh_ctrl_trq_NMM=global, RFootCnt=global, RLLoad=global, RLat_ctrl_trq=global, RLength=global, Ralpha=global, RdLength=global, Rdalpha=global, Rdgamma=global, Rgamma=global, Rphi12=global, Rphi23=global, Rshin_ctrl_trq=global, Rshin_ctrl_trq_NMM=global, RtauB=global, RtauF=global, Rthigh_ctrl_trq=global, Rthigh_ctrl_trq_NMM=global, b_SwLeg=global, b_inSw=global, dq=global, k_L=global, k_R=global, kinSw_BackFront=global, nm_Torque=global, q=global
  wires:
  [q] -> Robot-to-NMM Interface/1(q_discrete [rad] x13)
  [dq] -> Robot-to-NMM Interface/2(dq_discrete [rad/2] x13)
  Robot-to-NMM Interface/6(L Leg Load [bw]) -> [LLLoad]
  Robot-to-NMM Interface/5(R Leg Load [bw]) -> [RLLoad]
  Robot-to-NMM Interface/10(L Alpha [rad]) -> [Lalpha]
  Robot-to-NMM Interface/9(R Alpha [rad]) -> [Ralpha]
  Robot-to-NMM Interface/14(L Leg Length [m]) -> [LLength]
  Robot-to-NMM Interface/13(R Leg Length [m]) -> [RLength]
  Robot-to-NMM Interface/7(R Contact [0/1]) -> [RFootCnt]
  Robot-to-NMM Interface/8(L Contact [0/1]) -> [LFootCnt]
  Robot-to-NMM Interface/4(L_tau_front_meas [Nm]) -> [LtauF]
  Robot-to-NMM Interface/3(L_tau_back_meas [Nm]) -> [LtauB]
  Robot-to-NMM Interface/2(R_tau_front_meas [Nm]) -> [RtauF]
  Robot-to-NMM Interface/1(R_tau_back_meas [Nm]) -> [RtauB]
  Robot-to-NMM Interface/17(R virtual knee angle [rad]) -> [Rphi12]
  Robot-to-NMM Interface/18(R virtual hip angle [rad]) -> [Rphi23]
  Robot-to-NMM Interface/19(L virtual knee angle [rad]) -> [Lphi12]
  Robot-to-NMM Interface/20(L virtual hip angle [rad]) -> [Lphi23]
  Robot-to-NMM Interface/22(L Jacobian Constant (k)) -> [k_L]
  Robot-to-NMM Interface/21(R Jacobian Constant (k)) -> [k_R]
  Robot-to-NMM Interface/11(R dAlpha [rad/s]) -> [Rdalpha]
  Robot-to-NMM Interface/12(L dAlpha [rad/s]) -> [Ldalpha]
  Robot-to-NMM Interface/23(Rgamma [rad]) -> [Rgamma]
  Robot-to-NMM Interface/24(Lgamma [rad]) -> [Lgamma]
  Robot-to-NMM Interface/25(Rdgamma [rad]) -> [Rdgamma]
  Robot-to-NMM Interface/26(Ldgamma [rad]) -> [Ldgamma]
  Robot-to-NMM Interface/15(R Leg Length Velocity [m/s]) -> [RdLength]
  Robot-to-NMM Interface/16(L Leg Length Velocity [m/s]) -> [LdLength]
  Virtual Neuromuscular Control/1(RtauB_des [Nm]) -> [Rshin_ctrl_trq_NMM]  "Rshin"
  Virtual Neuromuscular Control/2(RtauF_des [Nm]) -> [Rthigh_ctrl_trq_NMM]  "Rthigh"
  Virtual Neuromuscular Control/3(LtauB_des [Nm]) -> [Lshin_ctrl_trq_NMM]  "Lshin"
  [Rshin_ctrl_trq_NMM] -> Mux7/1
  [Rthigh_ctrl_trq_NMM] -> Mux7/2
  [Lshin_ctrl_trq_NMM] -> Mux7/3
  [Lthigh_ctrl_trq_NMM] -> Mux7/4
  Demux3/4 -> [Lthigh_ctrl_trq]
  Demux3/3 -> [Lshin_ctrl_trq]
  Demux3/2 -> [Rthigh_ctrl_trq]
  Demux3/1 -> [Rshin_ctrl_trq]
  [Rshin_ctrl_trq] -> Mux/1  "Rshin"
  [Rthigh_ctrl_trq] -> Mux/2  "Rthigh"
  [RLat_ctrl_trq] -> Mux/3  "RLat"
  [Lshin_ctrl_trq] -> Mux/4  "Lshin"
  [Lthigh_ctrl_trq] -> Mux/5  "Lthigh"
  [LLat_ctrl_trq] -> Mux/6  "LLat"
  Mux/1 -> Add Limit Avoidance PD Torques/1(tau_des [Nm] x6)
  Lateral Motor Control/2(tau_lateral_L) -> [LLat_ctrl_trq]
  Lateral Motor Control/1(tau_lateral_R) -> [RLat_ctrl_trq]
  Constant/1 -> GRF XYZ estimates [N N N]/1
  q [rad] x13/1 -> [q]
  dq [rad/s] x13/1 -> [dq]
  Virtual Neuromuscular Control/4(LtauF_des [Nm]) -> [Lthigh_ctrl_trq_NMM]  "Lthigh"
  Mux7/1 -> Demux3/1
  [Ralpha] -> kinematic swing leg controller/4(Ralpha [rad])
  [Lalpha] -> kinematic swing leg controller/5(Lalpha [rad])
  [RFootCnt] -> kinematic swing leg controller/2(Rstance [1/0])
  [LFootCnt] -> kinematic swing leg controller/3(Lstance [1/0])
  [RLength] -> kinematic swing leg controller/6(Rlength [m])
  [LLength] -> kinematic swing leg controller/7(Llength [m])
  kinematic swing leg controller/1(Back/Front Motor Torque [Nm Nm]) -> [kinSw_BackFront]
  kinematic swing leg controller/3(SwLeg (right/left) [1/0]) -> [b_SwLeg]
  kinematic swing leg controller/2(inSw [1/0]) -> [b_inSw]
  Add Limit Avoidance PD Torques/1(tau_des w/PD [Nm] x6) -> [nm_Torque]
  [kinSw_BackFront] -> command routing/2(kinSw_command)
  [nm_Torque] -> command routing/1(nm_command)
  [b_inSw] -> command routing/3(inSwing [1/0])
  [b_SwLeg] -> command routing/4(SwLeg (right/left) [1/0])
  command routing/3(Force / Position Control [1/0] x4) -> Force / Position Control [1/0] x4/1
  [Rdgear_shin] -> Mux4/2
  [Rdgear_thigh] -> Mux1/2
  [Rgear_shin] -> Mux4/1
  [Rgear_thigh] -> Mux1/1
  [Lgear_shin] -> Mux2/1
  [Ldgear_shin] -> Mux2/2
  [Lgear_thigh] -> Mux3/1
  [Ldgear_thigh] -> Mux3/2
  Mux1/1 -> kinematic swing leg controller/9(RFront Gear [rad rad/s])
  Mux4/1 -> kinematic swing leg controller/8(RBack Gear [rad rad/s])
  Mux2/1 -> kinematic swing leg controller/10(LBack Gear [rad rad/s])
  Mux3/1 -> kinematic swing leg controller/11(LFront Gear [rad rad/s])
  command routing/1(Motor Torque Command [Nm] x6) -> Motor Torque Command [Nm] x6/1
  command routing/2(SEA Torque Velocity Command [Nm] x4) -> SEA Torque Velocity Command [Nm] x4/1
  Clock/1 -> Relational Operator/1
  Constant1/1 -> Relational Operator/2
  Relational Operator/1 -> kinematic swing leg controller/1(Ctrl On [1/0])
  [theta] -> kinematic swing leg controller/12(theta [rad])
  [kinSw_alpha_start] -> kinematic swing leg controller/13(alpha_init)
  [kinSw_alpha_tgt] -> kinematic swing leg controller/14(alpha_tgt [rad])
  [M4_G] -> command routing/5(M4_G)
  [kinSw_gH_tgt] -> kinematic swing leg controller/15(gH_tgt [m])
  [kinSw_gClr_tgt] -> kinematic swing leg controller/16(gclr_tgt [m])

== system atrias_HW_boom_nmSt_kinSw_v4/Control/Control Switch ==
  note: Switch Ctrl
  Pose Comm [Nm] x6 : Inport
  Pose Comm [Nm] x4 : Inport  Port=2
  Pose Comm [1/0] x4 : Inport  Port=3
  NM Comm [Nm] x6 : Inport  Port=4
  NM Comm [Nm] x4 : Inport  Port=5
  NM Comm [1/0] x4 : Inport  Port=6
  Constant2 : Constant  Value=flag_CtrlMode
  Demux1 : Demux  Outputs=2
  Multiport Switch : MultiPortSwitch  DataPortOrder=Zero-based contiguous  Inputs=2
  Multiport Switch1 : MultiPortSwitch  DataPortOrder=Zero-based contiguous  Inputs=2
  Mux : Mux  Inputs=2
  Mux1 : Mux  Inputs=2
  Motor Torque Command [Nm] x6 : Outport  OutputWhenDisabled=reset  InitialOutput=[0 0 0 0 0 0]
  SEA Torque Velocity Command [Nm] x4 : Outport  Port=2  OutputWhenDisabled=reset  InitialOutput=[0 0 0 0 0 0]
  Force / Position Control [1/0] x4 : Outport  Port=3  OutputWhenDisabled=reset  InitialOutput=[0 0 0 0 0 0]
  wires:
  Constant2/1 -> Multiport Switch1/1, Multiport Switch/1
  Mux/1 -> Multiport Switch/2
  Mux1/1 -> Multiport Switch/3
  Multiport Switch/1 -> Demux1/1
  Demux1/1 -> Motor Torque Command [Nm] x6/1
  Demux1/2 -> SEA Torque Velocity Command [Nm] x4/1
  Pose Comm [1/0] x4/1 -> Multiport Switch1/2
  NM Comm [1/0] x4/1 -> Multiport Switch1/3
  Multiport Switch1/1 -> Force / Position Control [1/0] x4/1
  Pose Comm [Nm] x6/1 -> Mux/1
  Pose Comm [Nm] x4/1 -> Mux/2
  NM Comm [Nm] x6/1 -> Mux1/1
  NM Comm [Nm] x4/1 -> Mux1/2

== system atrias_HW_boom_nmSt_kinSw_v4/Control/Poser ==
  note: ATRIAS Poser (on Air)
  Mux{5..6,8..9,11} (5 alike) : Mux  Inputs=2
  Subsystem : Subsystem
  Motor Torque Command [Nm] x6 : Outport  OutputWhenDisabled=reset  InitialOutput=[0 0 0 0 0 0]
  SEA Torque Velocity Command [Nm] x4 : Outport  Port=2  OutputWhenDisabled=reset  InitialOutput=[0 0 0 0 0 0]
  Force / Position Control [1/0] x4 : Outport  Port=3  OutputWhenDisabled=reset  InitialOutput=[0 0 0 0 0 0]
  wires:
  [poser_RLegLen] -> Subsystem/1(R legL)
  [Rdgear_shin] -> Mux9/2
  [Rdgear_thigh] -> Mux5/2
  [Rgear_shin] -> Mux9/1
  [Rgear_thigh] -> Mux5/1
  [Lgear_shin] -> Mux6/1
  [Ldgear_shin] -> Mux6/2
  [Lgear_thigh] -> Mux8/1
  [Ldgear_thigh] -> Mux8/2
  Mux5/1 -> Subsystem/6(R Front Gear)
  Mux9/1 -> Subsystem/5(R BackGear)
  Mux6/1 -> Subsystem/7(L BackGear)
  Mux8/1 -> Subsystem/8(L Front Gear)
  [poser_RLegAng] -> Subsystem/2(R phi)
  [poser_LLegLen] -> Subsystem/3(L legL)
  [poser_LLegAng] -> Subsystem/4(L phi)
  [RLat_ctrl_trq] -> Mux11/1
  [LLat_ctrl_trq] -> Mux11/2
  Mux11/1 -> Subsystem/9(Lateral Torque Command [Nm Nm])
  Subsystem/1(Motor Torque Command [Nm] x6) -> Motor Torque Command [Nm] x6/1
  Subsystem/2(SEA Torque Velocity Command [Nm] x4) -> SEA Torque Velocity Command [Nm] x4/1
  Subsystem/3(Force / Position Control [1/0] x4) -> Force / Position Control [1/0] x4/1

== system atrias_HW_boom_nmSt_kinSw_v4/Control/Tunable Control Parameters ==
  note: main controller
  note: intial poser
  tunable inputs : Inport
  Constant1 : Constant  Value=St_PreSHFL
  Constant10 : Constant  Value=TrCtrlPar
  Constant13 : Constant  Value=St_loffBFSH_VAS
  Constant14 : Constant  Value=St_LGainBFSH_VAS
  Constant15 : Constant  Value=St_loffBFSH
  Constant16 : Constant  Value=St_LGain_BFSH
  Constant17 : Constant  Value=St_SGainCGLU_HFL
  Constant19 : Constant  Value=St_SGainCHAM_HFL
  Constant2 : Constant  Value=LLCtrlPar
  Constant21 : Constant  Value=St_SGainGLU_HAM
  Constant22 : Constant  Value=St_SGainCHFL_GLU
  Constant23 : Constant  Value=St_SGainCRF_GLU
  Constant24 : Constant  Value=pi/2
  Constant3 : Constant  Value=St_PreSGLU
  Constant4 : Constant  Value=St_PreSHAM
  Constant5 : Constant  Value=St_PreSRF
  Constant6 : Constant  Value=FPCtrlPar
  Constant7 : Constant  Value=St_PreSVAS
  Constant8 : Constant  Value=St_PreSBFSH
  Constant9 : Constant  Value=SwCtrlPar
  Demux1 : Demux  Outputs=13
  Gain : Gain  Gain=1/FmaxVAS
  Gain{1..5} (5 alike) : Gain  Gain=pi/180
  Mux : Mux  Inputs=21
  Sum : Sum  Inputs=|++
  Sum1 : Sum  Inputs=|++
  tag scope: FPCtrlPar=global, LLCtrlPar=global, M4_G=global, StCtrlPar=global, SwCtrlPar=global, TrCtrlPar=global, kinSw_alpha_start=global, kinSw_alpha_tgt=global, kinSw_gClr_tgt=global, kinSw_gH_tgt=global, poser_LLegAng=global, poser_LLegLen=global, poser_RLegAng=global, poser_RLegLen=global, theta0=global
  wires:
  Constant6/1 -> [FPCtrlPar]
  Constant10/1 -> [TrCtrlPar]
  Constant9/1 -> [SwCtrlPar]
  Constant2/1 -> [LLCtrlPar]
  [tune_M3_0] -> Gain1/1
  [tune_M1_G] -> Gain/1
  Mux/1 -> [StCtrlPar]
  Gain1/1 -> [theta0]
  [poser_RLegLen] -> [poser_RLegLen]
  Sum/1 -> [poser_RLegAng]
  [poser_LLegLen] -> [poser_LLegLen]
  Sum1/1 -> [poser_LLegAng]
  [tune_kinSw_alpha_start] -> Gain4/1
  [tune_kinSw_alpha_tgt] -> Gain5/1
  Gain4/1 -> [kinSw_alpha_start]
  Gain5/1 -> [kinSw_alpha_tgt]
  [tune_kinSw_gH_tgt] -> [kinSw_gH_tgt]
  [tune_kinSw_gClr_tgt] -> [kinSw_gClr_tgt]
  [poser_RLegAlp] -> Gain3/1
  [poser_LLegAlp] -> Gain2/1
  Gain2/1 -> Sum1/1
  Gain3/1 -> Sum/1
  Constant24/1 -> Sum/2, Sum1/2
  Constant1/1 -> Mux/1
  Constant3/1 -> Mux/2
  Constant4/1 -> Mux/3
  Constant5/1 -> Mux/4
  Constant7/1 -> Mux/5
  Constant8/1 -> Mux/6
  Gain/1 -> Mux/7
  Constant13/1 -> Mux/8
  Constant14/1 -> Mux/9
  Constant15/1 -> Mux/10
  Constant16/1 -> Mux/11
  [tune_M3_P] -> Mux/14, Mux/12
  [tune_M3_D] -> Mux/15, Mux/13
  Constant21/1 -> Mux/21, Mux/16
  Constant17/1 -> Mux/17
  Constant19/1 -> Mux/18
  Constant22/1 -> Mux/19
  Constant23/1 -> Mux/20
  Demux1/1 -> [tune_M1_G]
  Demux1/2 -> [tune_M3_0]
  Demux1/3 -> [tune_M3_P]
  Demux1/4 -> [tune_M3_D]
  Demux1/6 -> [tune_kinSw_alpha_start]
  Demux1/7 -> [tune_kinSw_alpha_tgt]
  Demux1/8 -> [tune_kinSw_gH_tgt]
  Demux1/9 -> [tune_kinSw_gClr_tgt]
  Demux1/12 -> [poser_LLegLen]
  Demux1/13 -> [poser_LLegAlp]
  Demux1/10 -> [poser_RLegLen]
  Demux1/11 -> [poser_RLegAlp]
  Demux1/5 -> [tune_M4_G]
  tunable inputs/1 -> Demux1/1
  [tune_M4_G] -> [M4_G]

== system atrias_HW_boom_nmSt_kinSw_v4/Control/Actuator Control/Activate SEA Control ==
  SEA Control Signal [Nm] x4 : Inport
  "SEA on/off [1/0] x4 " : Inport  Port=2
  Torque Signal [Nm] x4 : Inport  Port=3
  Demux : Demux
  Demux2 : Demux
  Demux3 : Demux
  Mux6 : Mux
  Switch{,1..3} (4 alike) : Switch  Criteria=u2 ~= 0
  Torque Command [Nm] x4 : Outport
  wires:
  Demux2/2 -> Switch1/3
  Demux2/1 -> Switch/3
  Demux/1 -> Switch/1
  Switch/1 -> Mux6/1
  Switch1/1 -> Mux6/2
  Switch3/1 -> Mux6/4
  Demux3/1 -> Switch/2
  Mux6/1 -> Torque Command [Nm] x4/1
  Demux3/3 -> Switch2/2
  Demux3/2 -> Switch1/2
  Demux/3 -> Switch2/1
  Switch2/1 -> Mux6/3
  Demux/4 -> Switch3/1
  Demux2/4 -> Switch3/3
  Demux3/4 -> Switch3/2
  Demux/2 -> Switch1/1
  Demux2/3 -> Switch2/3
  SEA Control Signal [Nm] x4/1 -> Demux/1
  "SEA on/off [1/0] x4 "/1 -> Demux3/1
  Torque Signal [Nm] x4/1 -> Demux2/1

== system atrias_HW_boom_nmSt_kinSw_v4/Control/Actuator Control/Antiresonance Compensation ==
  Torque : Inport
  Notch Filter (Flight) : DiscreteTransferFcn  Numerator=[K_notch_f1 K_notch_f1*A1_notch_f1 K_notch_f1*A2_notch_f1]  Denominator=[1 B1_notch_f1 B2_notch_f1]  SampleTime=sample_time
  Filtered Torque : Outport
  wires:
  Torque/1 -> Notch Filter (Flight)/1
  Notch Filter (Flight)/1 -> Filtered Torque/1

== system atrias_HW_boom_nmSt_kinSw_v4/Control/Actuator Control/SEA Control Toggle ==
  enable : Inport
  tau_measured : Inport  Port=2
  tau_cmd : Inport  Port=3
  Abs : Abs
  Abs1 : Abs
  But Commanding a Small Torque? : simulink/Logic and Bit Operations/Compare To Constant  relop=<  const=sea_control_torque_cmd_small_threshold  OutDataTypeStr=boolean
  Logical Operator1 : Logic  AllPortsSameDT=off  OutDataTypeStr=boolean
  Logical Operator2 : Logic  Operator=NOT  AllPortsSameDT=off  OutDataTypeStr=boolean
  Logical Operator3 : Logic  AllPortsSameDT=off  OutDataTypeStr=boolean
  Logical Operator4 : Logic  AllPortsSameDT=off  OutDataTypeStr=boolean
  Measuring a Large Torque? (High Gains) : simulink/Logic and Bit Operations/Compare To Constant  relop=>=  const=loaded_unloaded_torque_threshold  OutDataTypeStr=boolean
  SEA Control on/off [1/0] : Outport
  wires:
  But Commanding a Small Torque?/1 -> Logical Operator1/2
  Logical Operator1/1 -> Logical Operator4/2
  tau_cmd/1 -> Abs/1
  Abs/1 -> But Commanding a Small Torque?/1
  tau_measured/1 -> Abs1/1
  Abs1/1 -> Measuring a Large Torque? (High Gains)/1
  Logical Operator3/1 -> SEA Control on/off [1/0]/1
  Logical Operator2/1 -> Logical Operator3/2
  Logical Operator4/1 -> Logical Operator2/1
  enable/1 -> Logical Operator4/1, Logical Operator3/1
  Measuring a Large Torque? (High Gains)/1 -> Logical Operator1/1

== system atrias_HW_boom_nmSt_kinSw_v4/Control/Actuator Control/SEA Controller (Torque) ==
  phi_load [rad] x4 : Inport
  phi_gear [rad] x4 : Inport  Port=2
  tau_des sagittal [Nm] x4 : Inport  Port=3
  dtau_des sagittal [Nm] x4 : Inport  Port=4
  dphi_load [rad/s] x4 : Inport  Port=5
  dphi_gear [rad/s] x4 : Inport  Port=6
  Abs : Abs
  Antiresonance Compensation : Subsystem
  Friction Compensation : Subsystem
  Loaded Unloaded Switch : Subsystem
  P gain ramp : Lookup_n-D  NumberOfTableDimensions=1  BreakpointsForDimension1=gain_nodes_sea_torque  Table=kp_sea_torque  InternalRulePriority=Speed  RndMeth=Simplest  InputSameDT=on
  Product : Product  SampleTime=sample_time  RndMeth=Zero
  Product2 : Product  RndMeth=Zero
  Spring Stiffness : Gain  Gain=k_sea
  Spring Stiffness 1 : Gain  Gain=k_sea
  Sum1 : Sum  Inputs=-+|
  Sum10 : Sum  Inputs=|++
  Sum2 : Sum  Inputs=|+-
  Sum3 : Sum  Inputs=++|
  Sum5 : Sum  Inputs=|+-
  Sum6 : Sum  Inputs=-+|
  Sum7 : Sum  Inputs=+|+
  Torque Limiter (outside) 1 : Saturate  UpperLimit=max_sagittal_loaded_torque  LowerLimit=-max_sagittal_loaded_torque
      settings: AttributesFormatString=Hi: %<UpperLimit>\nLo: %<LowerLimit>
  Torque Limiter (outside) 3 : Saturate  UpperLimit=max_sagittal_unloaded_torque  LowerLimit=-max_sagittal_unloaded_torque
      settings: AttributesFormatString=Hi: %<UpperLimit>\nLo: %<LowerLimit>
  Torque Threshold : simulink/Logic and Bit Operations/Compare To Constant  relop=>=  const=loaded_unloaded_torque_threshold  OutDataTypeStr=boolean
  critical damping : Subsystem
  tau_cmd sagittal [Nm] x4 : Outport
  tau_measured [Nm] x4 : Outport  Port=2
  wires:
  Product2/1 -> Sum7/2
  Sum2/1 -> Product2/2
  Sum5/1 -> Product/2
  dphi_gear [rad/s] x4/1 -> Friction Compensation/1(Motor Velocity [rad/s]), Sum6/2
  dphi_load [rad/s] x4/1 -> Sum6/1
  Spring Stiffness 1/1 -> Sum2/2
  Sum6/1 -> Spring Stiffness 1/1
  dtau_des sagittal [Nm] x4/1 -> Sum2/1
  tau_des sagittal [Nm] x4/1 -> Sum5/1
  phi_gear [rad] x4/1 -> Sum1/2
  phi_load [rad] x4/1 -> Sum1/1
  Sum1/1 -> Spring Stiffness/1
  Spring Stiffness/1 -> Sum3/1, Sum5/2, Abs/1, tau_measured [Nm] x4/1
  Sum10/1 -> Antiresonance Compensation/1(Torque), Torque Limiter (outside) 1/1
  P gain ramp/1 -> critical damping/1(p gain), Product/1
  Product/1 -> Sum7/1
  Sum7/1 -> Sum3/2
  Torque Limiter (outside) 1/1 -> Loaded Unloaded Switch/1(Loaded Signal)
  Torque Limiter (outside) 3/1 -> Loaded Unloaded Switch/2(Unloaded Signal)
  Antiresonance Compensation/1(Filtered Torque) -> Torque Limiter (outside) 3/1
  Friction Compensation/1(Friction Compensation [Nm]) -> Sum10/2
  Loaded Unloaded Switch/1(Signal) -> tau_cmd sagittal [Nm] x4/1
  Torque Threshold/1 -> Loaded Unloaded Switch/3(Loaded/Unloaded [1/0] x4)
  Abs/1 -> P gain ramp/1, Torque Threshold/1
  Sum3/1 -> Sum10/1
  critical damping/1(d gain) -> Product2/1

== system atrias_HW_boom_nmSt_kinSw_v4/Control/Behavior Control/Add Limit Avoidance PD Torques ==
  tau_des [Nm] x6 : Inport
  Mux4 : Mux  Inputs=2
  Selector2 : Selector  InputPortWidth=6  Indices=[1 2 4 5]
  Selector3 : Selector  InputPortWidth=6  Indices=[3 6]
  Selector8 : Selector  InputPortWidth=6  Indices=[1 2 5 3 4 6]
  Zero-Order Hold (1kHz)4 : ZeroOrderHold  SampleTime=sample_time
  mechanical limit avoidance : Subsystem
  tau_des w/PD [Nm] x6 : Outport
  wires:
  Zero-Order Hold (1kHz)4/1 -> Selector2/1, Selector3/1
  tau_des [Nm] x6/1 -> Zero-Order Hold (1kHz)4/1
  Selector8/1 -> tau_des w/PD [Nm] x6/1
  Mux4/1 -> Selector8/1
  Selector3/1 -> Mux4/2
  Selector2/1 -> mechanical limit avoidance/1(tau_des [Nm]x4)
  mechanical limit avoidance/1(tau_des + pd [Nm]x4) -> Mux4/1

== system atrias_HW_boom_nmSt_kinSw_v4/Control/Behavior Control/Lateral Motor Control ==
  note: PD + Buckling Compensation
  Lateral Control1 : MATLAB Function  TreatAsAtomicUnit=on
  Left Lateral Torque Saturation : Saturate  UpperLimit=max_torque_lateral  LowerLimit=-max_torque_lateral
      settings: AttributesFormatString=Top: %<UpperLimit>\nBottom: %<LowerLimit>
  Right Lateral Torque Saturation : Saturate  UpperLimit=max_torque_lateral  LowerLimit=-max_torque_lateral
      settings: AttributesFormatString=Top: %<UpperLimit>\nBottom: %<LowerLimit>
  percent body weight : Gain  Gain=(m_total*g)
  percent body weight1 : Gain  Gain=(m_total*g)
  tau_lateral_R : Outport
  tau_lateral_L : Outport  Port=2
  wires:
  Lateral Control1/1(tau_r) -> Right Lateral Torque Saturation/1
  Lateral Control1/2(tau_l) -> Left Lateral Torque Saturation/1
  Right Lateral Torque Saturation/1 -> tau_lateral_R/1
  Left Lateral Torque Saturation/1 -> tau_lateral_L/1
  [Rphi_Lat] -> Lateral Control1/1(qLateralR)
  [Rdphi_Lat] -> Lateral Control1/2(dqLateralR)
  [Lphi_Lat] -> Lateral Control1/3(qLateralL)
  [Ldphi_Lat] -> Lateral Control1/4(dqLateralL)
  [RLLoad] -> percent body weight/1
  [LLLoad] -> percent body weight1/1
  percent body weight/1 -> Lateral Control1/5(F_leg_R)
  percent body weight1/1 -> Lateral Control1/6(F_leg_L)
